simulink model "simulink-for-setup"  (R2015b)
settings: Solver=VariableStepAuto  StartTime=0.0  StopTime=3  RelTol=1e-3
libraries: arduino_io_lib x4
settings Model: Creator=mctra  LastModifiedBy=mctra

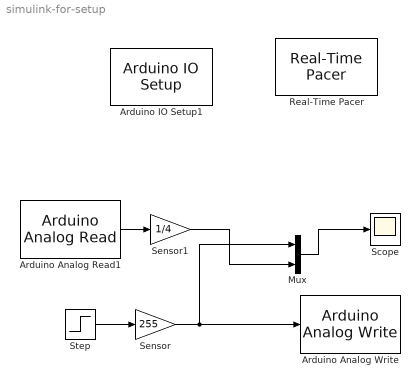
== system simulink-for-setup ==
  Arduino Analog Read1 : arduino_io_lib/Arduino Analog Read  arduinoVar=Temporary arduino variable: Arduino1  arduinoPin=0  T=0.2
  Arduino Analog Write : arduino_io_lib/Arduino Analog Write  arduinoVar=Temporary arduino variable: Arduino1  arduinoPin=9  T=0.2
  Arduino IO Setup1 : arduino_io_lib/Arduino IO Setup  Priority=3  arduinoVar=Temporary arduino variable: Arduino1  workspaceVarName=a  comPort=COM1
  Mux : Mux  Inputs=2
  Real-Time Pacer : arduino_io_lib/Real-Time Pacer  simTimePerRealTime=1
  Scope : Scope
  Sensor : Gain  Gain=255
  Sensor1 : Gain  Gain=1/4
  Step : Step  SampleTime=0
  wires:
  Arduino Analog Read1/1 -> Sensor1/1
  Step/1 -> Sensor/1
  Mux/1 -> Scope/1
  Sensor/1 -> Mux/1, Arduino Analog Write/1
  Sensor1/1 -> Mux/2
